simulink library "Gradiantel_Force"  (R2020b)
settings: Solver=VariableStepAuto  StartTime=0.0  StopTime=10.0  RelTol=1e-3
values from neighbouring files (symbols this model uses):
  g = 9.81    [Projektskript.m]    (also in init.m)
  m = 2000    [Projektskript.m]    (also in init.m)
settings Model: Creator=janbantle  LastModifiedBy=Johnathy

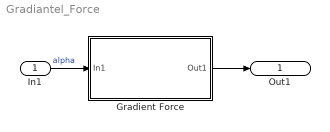
== system Gradiantel_Force ==
  In1 : Inport
  Gradient Force : Subsystem
  Out1 : Outport
  wires:
  In1/1 -> Gradient Force/1(In1)  "alpha"
  Gradient Force/1(Out1) -> Out1/1

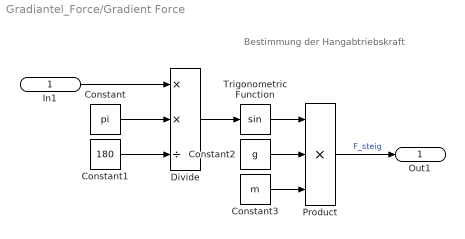
== system Gradiantel_Force/Gradient Force ==
  note: Bestimmung der Hangabtriebskraft
  In1 : Inport
  Constant : Constant  Value=pi
  Constant1 : Constant  Value=180
  Constant2 : Constant  Value=g
  Constant3 : Constant  Value=m
  Divide : Product  Inputs=**/
  Product : Product  Inputs=3
  Trigonometric Function : Trigonometry
  Out1 : Outport
  wires:
  Constant/1 -> Divide/2
  Trigonometric Function/1 -> Product/1
  In1/1 -> Divide/1
  Product/1 -> Out1/1  "F_steig"
  Constant1/1 -> Divide/3
  Divide/1 -> Trigonometric Function/1
  Constant2/1 -> Product/2
  Constant3/1 -> Product/3
